simulink model "Simulation"  (R2022b)
settings: Solver=VariableStepAuto  StartTime=0.0  StopTime=300  RelTol=1e-3
values from neighbouring files (symbols this model uses):
  At = 63.6    [LAB.m]
  K_q = 10    [LAB.m]
  point = [14, 14]    [LAB.m]
  u_1_init = double(solve(eqs_solve(1)==0,u_1))    [LAB.m]
  u_2_init = double(solve(eqs_solve(2)==0,u_2))    [LAB.m]
settings Model: Creator=danisode  LastModifiedBy=soder

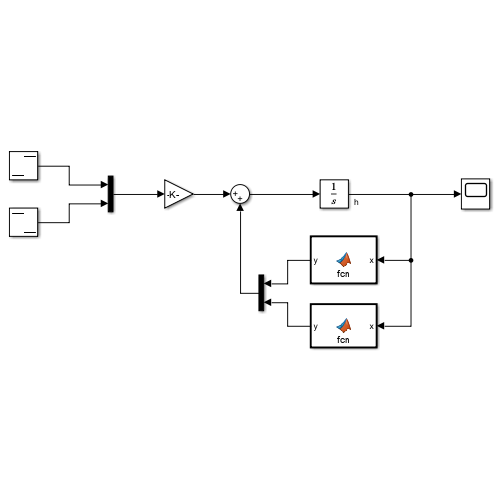
[thumbnail: Simulink's stored preview of the top-level diagram]
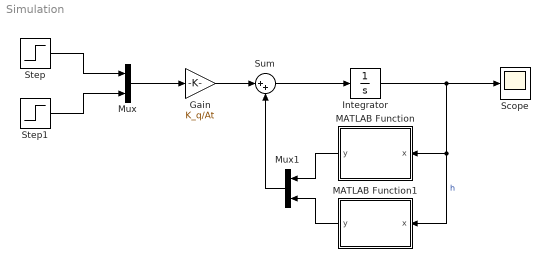
== system Simulation ==
  Gain : Gain  Gain=K_q/At
  Integrator : Integrator  InitialCondition=point
  MATLAB Function : MATLAB Function  TreatAsAtomicUnit=on
  MATLAB Function1 : MATLAB Function  TreatAsAtomicUnit=on
  Mux : Mux  Inputs=2
  Mux1 : Mux  Inputs=2
  Scope : Scope
  Step : Step  Time=0.1  Before=u_1_init  After=5  SampleTime=15
  Step1 : Step  Before=u_2_init  After=3  SampleTime=15
  Sum : Sum  Inputs=|++
  wires:
  Step/1 -> Mux/1
  Step1/1 -> Mux/2
  Mux/1 -> Gain/1
  Gain/1 -> Sum/1
  Sum/1 -> Integrator/1
  Integrator/1 -> MATLAB Function1/1(x), MATLAB Function/1(x), Scope/1  "h"
  MATLAB Function1/1(y) -> Mux1/2
  MATLAB Function/1(y) -> Mux1/1
  Mux1/1 -> Sum/2

== matlab function Simulation/MATLAB Function1 ==
  data: x input; y output
function y = fcn(x)
h_1 = x(1);
h_2 = x(2);
y = (5*h_1)/53 - (5*h_2)/53 - (119*218^(1/2)*h_2^(1/2))/10600;

== matlab function Simulation/MATLAB Function ==
  data: x input; y output
function y = fcn(x)
h_1 = x(1);
h_2 = x(2);
y = (5*h_2)/53 - (5*h_1)/53 - (119*218^(1/2)*h_1^(1/2))/10600;
